simulink model "probThree"  (R2020b)
settings: Solver=ode45  StartTime=0.0  StopTime=10.0  MaxStep=0.001  RelTol=1e-3
model workspace (MAT data in the model file):
  h2r = 5
settings Model: Creator='Z'ome  LastModifiedBy='Z'ome

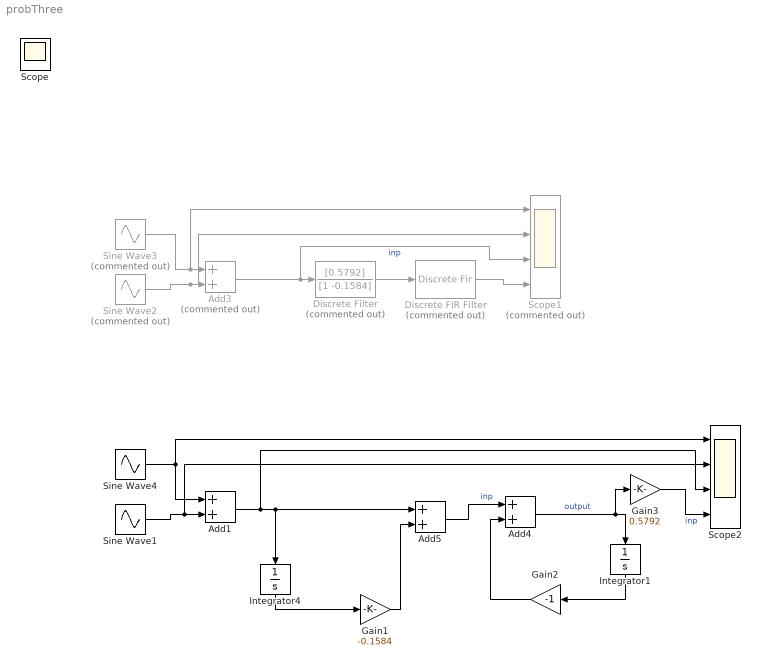
== system probThree ==
  Add1 : Sum
  Add3 : Sum  Commented=on
  Add4 : Sum
  Add5 : Sum
  Discrete FIR Filter : DiscreteFir  Commented=on  Coefficients=[1 -1]
  Discrete Filter : DiscreteFilter  Commented=on  Numerator=[0.5792]  Denominator=[1 -0.1584]
  Gain1 : Gain  Gain=-0.1584
  Gain2 : Gain  Gain=-1
  Gain3 : Gain  Gain=0.5792
  Integrator1 : Integrator
  Integrator4 : Integrator
  Scope1 : Scope  Commented=on  NumInputPorts=4
  Scope2 : Scope  NumInputPorts=4
  Sine Wave1 : Sin  Frequency=100  SampleTime=0
  Sine Wave2 : Sin  Commented=on  Frequency=100*h2r  SampleTime=0
  Sine Wave3 : Sin  Commented=on  Frequency=1/5*h2r  SampleTime=0
  Sine Wave4 : Sin  SampleTime=0
  Scope : Scope
  wires:
  Discrete Filter/1 -> Discrete FIR Filter/1
  Add3/1 -> Scope1/3, Discrete Filter/1  "inp"
  Sine Wave3/1 -> Scope1/1, Add3/1
  Sine Wave2/1 -> Scope1/2, Add3/2
  Discrete FIR Filter/1 -> Scope1/4
  Sine Wave1/1 -> Add1/2, Scope2/2
  Sine Wave4/1 -> Add1/1, Scope2/1
  Add1/1 -> Add5/1, Integrator4/1, Scope2/3
  Integrator1/1 -> Gain2/1
  Gain2/1 -> Add4/2
  Add4/1 -> Gain3/1, Integrator1/1  "output"
  Add5/1 -> Add4/1  "inp"
  Integrator4/1 -> Gain1/1
  Gain1/1 -> Add5/2
  Gain3/1 -> Scope2/4  "inp"
